simulink model "DeadTimevsTimeConstant"  (R2018b)
settings: Solver=FixedStepAuto  StartTime=0.0  StopTime=60  FixedStep=0.01  RelTol=1e-3
libraries: simulink x2
settings Model: Creator=Trips  LastModifiedBy=Trips

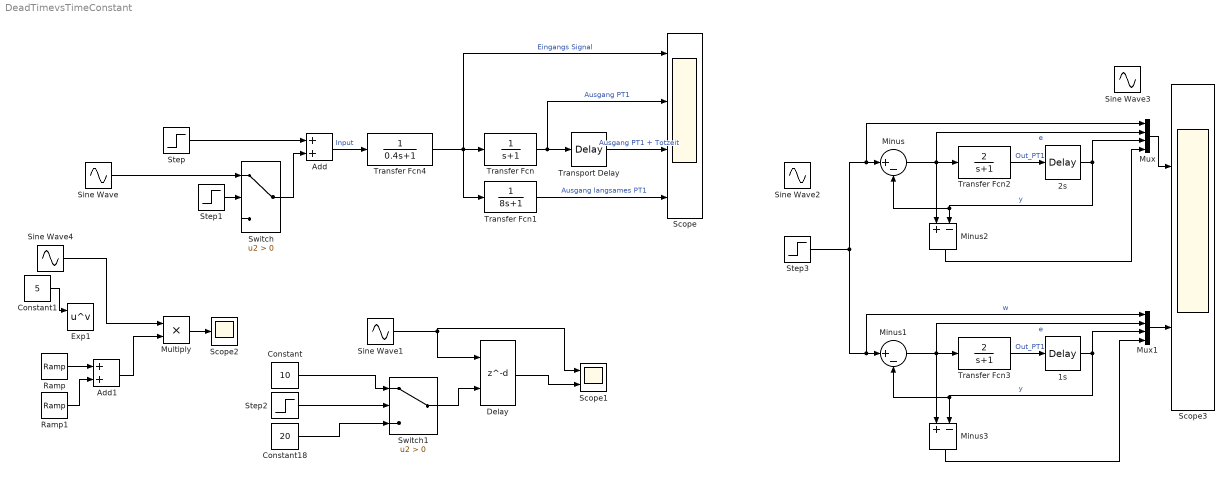
== system DeadTimevsTimeConstant ==
  "1s " : TransportDelay
  2s : TransportDelay  DelayTime=2
  Add : Sum
  Add1 : Sum
  Constant : Constant  Value=10
  Constant1 : Constant  Value=5
  Constant18 : Constant  Value=20
  Delay : Delay  DelayLengthSource=Input port  DelayLength=600  DelayLengthUpperLimit=800
      settings: InputPortMap=u0,p1
  Exp1 : Math  Operator=pow  SaturateOnIntegerOverflow=on
  Minus : Sum  Inputs=|+-
  Minus1 : Sum  Inputs=|+-
  Minus2 : Sum  Inputs=+-
  Minus3 : Sum  Inputs=+-
  Multiply : Product
  Mux : Mux
  Mux1 : Mux
  Ramp : simulink/Sources/Ramp  slope=0.1  start=30  InitialOutput=0
  Ramp1 : simulink/Sources/Ramp  slope=-0.1  start=40  InitialOutput=0
  Scope : Scope  NumInputPorts=4
  Scope1 : Scope  NumInputPorts=2
  Scope2 : Scope
  Scope3 : Scope  NumInputPorts=2
  Sine Wave : Sin  Frequency=0.5  Phase=-30*0.5  SampleTime=0
  Sine Wave1 : Sin  SampleTime=0
  Sine Wave2 : Sin  Frequency=0.5  SampleTime=0
  Sine Wave3 : Sin  Frequency=1.732  Phase=-2.5*1.732  SampleTime=0
  Sine Wave4 : Sin  Frequency=0.5  Phase=-30*0.5  SampleTime=0
  Step : Step  SampleTime=0
  Step1 : Step  Time=30  SampleTime=0
  Step2 : Step  Time=10  Before=1  After=0  SampleTime=0
  Step3 : Step  SampleTime=0
  Switch : Switch  Criteria=u2 > Threshold
  Switch1 : Switch  Criteria=u2 > Threshold
  Transfer Fcn : TransferFcn  Denominator=[1 1]
  Transfer Fcn1 : TransferFcn  Denominator=[8 1]
  Transfer Fcn2 : TransferFcn  Numerator=[2]  Denominator=[1 1]
  Transfer Fcn3 : TransferFcn  Numerator=[2]  Denominator=[1 1]
  Transfer Fcn4 : TransferFcn  Denominator=[0.4 1]
  Transport Delay : TransportDelay  DelayTime=1.5
  wires:
  Transfer Fcn/1 -> Scope/2, Transport Delay/1  "Ausgang PT1"
  Step/1 -> Add/1
  Transport Delay/1 -> Scope/3  "Ausgang PT1 + Totzeit"
  Add/1 -> Transfer Fcn4/1  "Input"
  Switch/1 -> Add/2
  Step1/1 -> Switch/2
  Transfer Fcn1/1 -> Scope/4  "Ausgang langsames PT1"
  Switch1/1 -> Delay/2
  Constant/1 -> Switch1/1
  Delay/1 -> Scope1/2
  Sine Wave1/1 -> Delay/1, Scope1/1
  Constant18/1 -> Switch1/3
  Step2/1 -> Switch1/2
  Transfer Fcn2/1 -> 2s/1  "Out_PT1"
  Minus/1 -> Minus2/1, Mux/2, Transfer Fcn2/1  "e"
  2s/1 -> Minus/2, Minus2/2, Mux/3  "y"
  Mux/1 -> Scope3/1
  Minus1/1 -> Minus3/1, Transfer Fcn3/1, Mux1/2  "e"
  Step3/1 -> Mux1/1, Minus1/1, Mux/1, Minus/1  "w"
  Transfer Fcn3/1 -> "1s "/1  "Out_PT1"
  Mux1/1 -> Scope3/2
  "1s "/1 -> Minus1/2, Minus3/2, Mux1/3  "y"
  Minus3/1 -> Mux1/4
  Minus2/1 -> Mux/4
  Transfer Fcn4/1 -> Transfer Fcn1/1, Scope/1, Transfer Fcn/1  "Eingangs Signal"
  Sine Wave/1 -> Switch/1
  Sine Wave4/1 -> Multiply/1
  Add1/1 -> Multiply/2
  Constant1/1 -> Exp1/1
  Multiply/1 -> Scope2/1
  Ramp/1 -> Add1/1
  Ramp1/1 -> Add1/2
